simulink subsystem "Plant"  (R2024b)
settings: Solver=VariableStepAuto  StartTime=0.0  StopTime=10.0  RelTol=1e-3
model mask{setup=launch_initial, switch_time=0, mu=Earth_planet.mu}
  mask prompts: setup "Setup Data"; switch_time "Gravity Switch Time"; mu "Gravitational Parameter"
libraries: vrlib x1
settings Model: Creator=cpero  LastModifiedBy=cpero

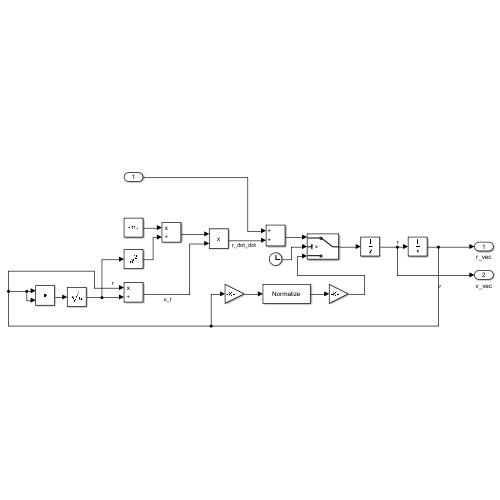
[thumbnail: Simulink's stored preview of the top-level diagram]
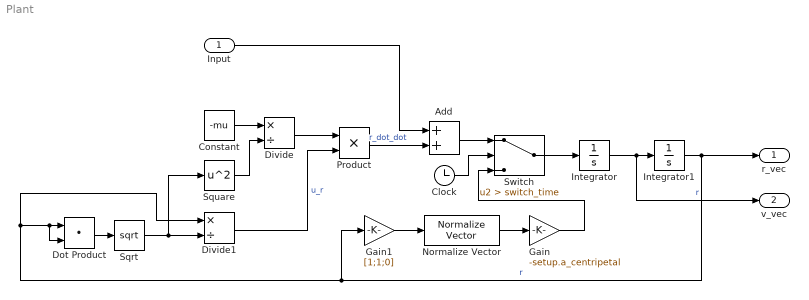
== system Plant ==
  Input : Inport
  Add : Sum
  Clock : Clock
  Constant : Constant  Value=-mu
  Divide : Product  Inputs=*/
  Divide1 : Product  Inputs=*/
  Dot Product : DotProduct  OutDataTypeStr=Inherit: Inherit via internal rule
  Gain : Gain  Gain=-setup.a_centripetal
  Gain1 : Gain  Gain=[1;1;0]
  Integrator : Integrator  InitialCondition=setup.v_initial
  Integrator1 : Integrator  InitialCondition=setup.r_initial
  Normalize Vector : vrlib/Utilities/Normalize Vector  maxzero=0
  Product : Product
  Sqrt : Sqrt
  Square : Math  Operator=square
  Switch : Switch  Criteria=u2 > Threshold  Threshold=switch_time  ZeroCross=off  SaturateOnIntegerOverflow=off  InputSameDT=off
  r_vec : Outport
  v_vec : Outport  Port=2
  wires:
  Integrator1/1 -> r_vec/1, Divide1/1, Dot Product/1, Dot Product/2, Gain1/1  "r"
  Divide1/1 -> Product/2  "u_r"
  Sqrt/1 -> Divide1/2, Square/1
  Divide/1 -> Product/1
  Square/1 -> Divide/2
  Dot Product/1 -> Sqrt/1
  Constant/1 -> Divide/1
  Product/1 -> Add/2  "r_dot_dot"
  Switch/1 -> Integrator/1
  Add/1 -> Switch/1
  Clock/1 -> Switch/2
  Normalize Vector/1 -> Gain/1
  Gain/1 -> Switch/3
  Gain1/1 -> Normalize Vector/1
  Integrator/1 -> Integrator1/1, v_vec/1  "r"
  Input/1 -> Add/1
